simulink model "signal_tranmission"  (R2024b)
settings: Solver=ode45  StartTime=0.0  StopTime=10  FixedStep=0.000125  RelTol=1e-3
libraries: dspfdesign x500, commchan3 x1
(part 3 of 7)

== system signal_tranmission/SSB Demod92 ==
  Input Signal : Inport
  Analog Filter Design1 : dspfdesign/Analog Filter Design  method=Butterworth  filttype=Lowpass  N=4  Wlo=5*2*pi  Whi=102*2*pi  Rp=2  Rs=40
  Balanced Modulator1 : Subsystem
  carrier signal : Sin  Frequency=468*2*pi  SampleTime=0
  Out1 : Outport
  wires:
  Analog Filter Design1/1 -> Out1/1
  Balanced Modulator1/1(DSBSC) -> Analog Filter Design1/1
  carrier signal/1 -> Balanced Modulator1/2(Carrier Signal)
  Input Signal/1 -> Balanced Modulator1/1(Input Signal)

== system signal_tranmission/SSB Demod93 ==
  Input Signal : Inport
  Analog Filter Design1 : dspfdesign/Analog Filter Design  method=Butterworth  filttype=Lowpass  N=4  Wlo=5*2*pi  Whi=102*2*pi  Rp=2  Rs=40
  Balanced Modulator1 : Subsystem
  carrier signal : Sin  Frequency=472*2*pi  SampleTime=0
  Out1 : Outport
  wires:
  Analog Filter Design1/1 -> Out1/1
  Balanced Modulator1/1(DSBSC) -> Analog Filter Design1/1
  carrier signal/1 -> Balanced Modulator1/2(Carrier Signal)
  Input Signal/1 -> Balanced Modulator1/1(Input Signal)

== system signal_tranmission/SSB Demod94 ==
  Input Signal : Inport
  Analog Filter Design1 : dspfdesign/Analog Filter Design  method=Butterworth  filttype=Lowpass  N=4  Wlo=5*2*pi  Whi=102*2*pi  Rp=2  Rs=40
  Balanced Modulator1 : Subsystem
  carrier signal : Sin  Frequency=476*2*pi  SampleTime=0
  Out1 : Outport
  wires:
  Analog Filter Design1/1 -> Out1/1
  Balanced Modulator1/1(DSBSC) -> Analog Filter Design1/1
  carrier signal/1 -> Balanced Modulator1/2(Carrier Signal)
  Input Signal/1 -> Balanced Modulator1/1(Input Signal)

== system signal_tranmission/SSB Demod95 ==
  Input Signal : Inport
  Analog Filter Design1 : dspfdesign/Analog Filter Design  method=Butterworth  filttype=Lowpass  N=4  Wlo=5*2*pi  Whi=102*2*pi  Rp=2  Rs=40
  Balanced Modulator1 : Subsystem
  carrier signal : Sin  Frequency=480*2*pi  SampleTime=0
  Out1 : Outport
  wires:
  Analog Filter Design1/1 -> Out1/1
  Balanced Modulator1/1(DSBSC) -> Analog Filter Design1/1
  carrier signal/1 -> Balanced Modulator1/2(Carrier Signal)
  Input Signal/1 -> Balanced Modulator1/1(Input Signal)

== system signal_tranmission/SSB Demod96 ==
  Input Signal : Inport
  Analog Filter Design1 : dspfdesign/Analog Filter Design  method=Butterworth  filttype=Lowpass  N=4  Wlo=5*2*pi  Whi=102*2*pi  Rp=2  Rs=40
  Balanced Modulator1 : Subsystem
  carrier signal : Sin  Frequency=484*2*pi  SampleTime=0
  Out1 : Outport
  wires:
  Analog Filter Design1/1 -> Out1/1
  Balanced Modulator1/1(DSBSC) -> Analog Filter Design1/1
  carrier signal/1 -> Balanced Modulator1/2(Carrier Signal)
  Input Signal/1 -> Balanced Modulator1/1(Input Signal)

== system signal_tranmission/SSB Demod97 ==
  Input Signal : Inport
  Analog Filter Design1 : dspfdesign/Analog Filter Design  method=Butterworth  filttype=Lowpass  N=4  Wlo=5*2*pi  Whi=102*2*pi  Rp=2  Rs=40
  Balanced Modulator1 : Subsystem
  carrier signal : Sin  Frequency=488*2*pi  SampleTime=0
  Out1 : Outport
  wires:
  Analog Filter Design1/1 -> Out1/1
  Balanced Modulator1/1(DSBSC) -> Analog Filter Design1/1
  carrier signal/1 -> Balanced Modulator1/2(Carrier Signal)
  Input Signal/1 -> Balanced Modulator1/1(Input Signal)

== system signal_tranmission/SSB Demod98 ==
  Input Signal : Inport
  Analog Filter Design1 : dspfdesign/Analog Filter Design  method=Butterworth  filttype=Lowpass  N=4  Wlo=5*2*pi  Whi=102*2*pi  Rp=2  Rs=40
  Balanced Modulator1 : Subsystem
  carrier signal : Sin  Frequency=492*2*pi  SampleTime=0
  Out1 : Outport
  wires:
  Analog Filter Design1/1 -> Out1/1
  Balanced Modulator1/1(DSBSC) -> Analog Filter Design1/1
  carrier signal/1 -> Balanced Modulator1/2(Carrier Signal)
  Input Signal/1 -> Balanced Modulator1/1(Input Signal)

== system signal_tranmission/SSB Demod99 ==
  Input Signal : Inport
  Analog Filter Design1 : dspfdesign/Analog Filter Design  method=Butterworth  filttype=Lowpass  N=4  Wlo=5*2*pi  Whi=102*2*pi  Rp=2  Rs=40
  Balanced Modulator1 : Subsystem
  carrier signal : Sin  Frequency=496*2*pi  SampleTime=0
  Out1 : Outport
  wires:
  Analog Filter Design1/1 -> Out1/1
  Balanced Modulator1/1(DSBSC) -> Analog Filter Design1/1
  carrier signal/1 -> Balanced Modulator1/2(Carrier Signal)
  Input Signal/1 -> Balanced Modulator1/1(Input Signal)

== system signal_tranmission/SSB Modulator ==
  Input Signal : Inport
  Analog Filter Design : dspfdesign/Analog Filter Design  method=Butterworth  filttype=Bandpass  N=4  Wlo=98*2*pi  Whi=102*2*pi  Rp=2  Rs=40
  Balanced Modulator : Subsystem
  carrier signal : Sin  Frequency=100*2*pi  SampleTime=0
  Out1 : Outport
  wires:
  carrier signal/1 -> Balanced Modulator/2(Carrier Signal)
  Balanced Modulator/1(DSBSC) -> Analog Filter Design/1
  Analog Filter Design/1 -> Out1/1
  Input Signal/1 -> Balanced Modulator/1(Input Signal)

== system signal_tranmission/SSB Modulator1 ==
  Input Signal : Inport
  Analog Filter Design : dspfdesign/Analog Filter Design  method=Butterworth  filttype=Bandpass  N=4  Wlo=102*2*pi  Whi=106*2*pi  Rp=2  Rs=40
  Balanced Modulator : Subsystem
  carrier signal : Sin  Frequency=104*2*pi  SampleTime=0
  Out1 : Outport
  wires:
  carrier signal/1 -> Balanced Modulator/2(Carrier Signal)
  Balanced Modulator/1(DSBSC) -> Analog Filter Design/1
  Analog Filter Design/1 -> Out1/1
  Input Signal/1 -> Balanced Modulator/1(Input Signal)

== system signal_tranmission/SSB Modulator10 ==
  Input Signal : Inport
  Analog Filter Design : dspfdesign/Analog Filter Design  method=Butterworth  filttype=Bandpass  N=4  Wlo=138*2*pi  Whi=142*2*pi  Rp=2  Rs=40
  Balanced Modulator : Subsystem
  carrier signal : Sin  Frequency=140*2*pi  SampleTime=0
  Out1 : Outport
  wires:
  carrier signal/1 -> Balanced Modulator/2(Carrier Signal)
  Balanced Modulator/1(DSBSC) -> Analog Filter Design/1
  Analog Filter Design/1 -> Out1/1
  Input Signal/1 -> Balanced Modulator/1(Input Signal)

== system signal_tranmission/SSB Modulator11 ==
  Input Signal : Inport
  Analog Filter Design : dspfdesign/Analog Filter Design  method=Butterworth  filttype=Bandpass  N=4  Wlo=142*2*pi  Whi=146*2*pi  Rp=2  Rs=40
  Balanced Modulator : Subsystem
  carrier signal : Sin  Frequency=144*2*pi  SampleTime=0
  Out1 : Outport
  wires:
  carrier signal/1 -> Balanced Modulator/2(Carrier Signal)
  Balanced Modulator/1(DSBSC) -> Analog Filter Design/1
  Analog Filter Design/1 -> Out1/1
  Input Signal/1 -> Balanced Modulator/1(Input Signal)

== system signal_tranmission/SSB Modulator12 ==
  Input Signal : Inport
  Analog Filter Design : dspfdesign/Analog Filter Design  method=Butterworth  filttype=Bandpass  N=4  Wlo=146*2*pi  Whi=150*2*pi  Rp=2  Rs=40
  Balanced Modulator : Subsystem
  carrier signal : Sin  Frequency=148*2*pi  SampleTime=0
  Out1 : Outport
  wires:
  carrier signal/1 -> Balanced Modulator/2(Carrier Signal)
  Balanced Modulator/1(DSBSC) -> Analog Filter Design/1
  Analog Filter Design/1 -> Out1/1
  Input Signal/1 -> Balanced Modulator/1(Input Signal)

== system signal_tranmission/SSB Modulator13 ==
  Input Signal : Inport
  Analog Filter Design : dspfdesign/Analog Filter Design  method=Butterworth  filttype=Bandpass  N=4  Wlo=150*2*pi  Whi=154*2*pi  Rp=2  Rs=40
  Balanced Modulator : Subsystem
  carrier signal : Sin  Frequency=152*2*pi  SampleTime=0
  Out1 : Outport
  wires:
  carrier signal/1 -> Balanced Modulator/2(Carrier Signal)
  Balanced Modulator/1(DSBSC) -> Analog Filter Design/1
  Analog Filter Design/1 -> Out1/1
  Input Signal/1 -> Balanced Modulator/1(Input Signal)

== system signal_tranmission/SSB Modulator14 ==
  Input Signal : Inport
  Analog Filter Design : dspfdesign/Analog Filter Design  method=Butterworth  filttype=Bandpass  N=4  Wlo=154*2*pi  Whi=158*2*pi  Rp=2  Rs=40
  Balanced Modulator : Subsystem
  carrier signal : Sin  Frequency=156*2*pi  SampleTime=0
  Out1 : Outport
  wires:
  carrier signal/1 -> Balanced Modulator/2(Carrier Signal)
  Balanced Modulator/1(DSBSC) -> Analog Filter Design/1
  Analog Filter Design/1 -> Out1/1
  Input Signal/1 -> Balanced Modulator/1(Input Signal)

== system signal_tranmission/SSB Modulator15 ==
  Input Signal : Inport
  Analog Filter Design : dspfdesign/Analog Filter Design  method=Butterworth  filttype=Bandpass  N=4  Wlo=158*2*pi  Whi=162*2*pi  Rp=2  Rs=40
  Balanced Modulator : Subsystem
  carrier signal : Sin  Frequency=160*2*pi  SampleTime=0
  Out1 : Outport
  wires:
  carrier signal/1 -> Balanced Modulator/2(Carrier Signal)
  Balanced Modulator/1(DSBSC) -> Analog Filter Design/1
  Analog Filter Design/1 -> Out1/1
  Input Signal/1 -> Balanced Modulator/1(Input Signal)

== system signal_tranmission/SSB Modulator16 ==
  Input Signal : Inport
  Analog Filter Design : dspfdesign/Analog Filter Design  method=Butterworth  filttype=Bandpass  N=4  Wlo=162*2*pi  Whi=166*2*pi  Rp=2  Rs=40
  Balanced Modulator : Subsystem
  carrier signal : Sin  Frequency=164*2*pi  SampleTime=0
  Out1 : Outport
  wires:
  carrier signal/1 -> Balanced Modulator/2(Carrier Signal)
  Balanced Modulator/1(DSBSC) -> Analog Filter Design/1
  Analog Filter Design/1 -> Out1/1
  Input Signal/1 -> Balanced Modulator/1(Input Signal)

== system signal_tranmission/SSB Modulator17 ==
  Input Signal : Inport
  Analog Filter Design : dspfdesign/Analog Filter Design  method=Butterworth  filttype=Bandpass  N=4  Wlo=166*2*pi  Whi=170*2*pi  Rp=2  Rs=40
  Balanced Modulator : Subsystem
  carrier signal : Sin  Frequency=168*2*pi  SampleTime=0
  Out1 : Outport
  wires:
  carrier signal/1 -> Balanced Modulator/2(Carrier Signal)
  Balanced Modulator/1(DSBSC) -> Analog Filter Design/1
  Analog Filter Design/1 -> Out1/1
  Input Signal/1 -> Balanced Modulator/1(Input Signal)

== system signal_tranmission/SSB Modulator18 ==
  Input Signal : Inport
  Analog Filter Design : dspfdesign/Analog Filter Design  method=Butterworth  filttype=Bandpass  N=4  Wlo=170*2*pi  Whi=174*2*pi  Rp=2  Rs=40
  Balanced Modulator : Subsystem
  carrier signal : Sin  Frequency=172*2*pi  SampleTime=0
  Out1 : Outport
  wires:
  carrier signal/1 -> Balanced Modulator/2(Carrier Signal)
  Balanced Modulator/1(DSBSC) -> Analog Filter Design/1
  Analog Filter Design/1 -> Out1/1
  Input Signal/1 -> Balanced Modulator/1(Input Signal)

== system signal_tranmission/SSB Modulator19 ==
  Input Signal : Inport
  Analog Filter Design : dspfdesign/Analog Filter Design  method=Butterworth  filttype=Bandpass  N=4  Wlo=174*2*pi  Whi=178*2*pi  Rp=2  Rs=40
  Balanced Modulator : Subsystem
  carrier signal : Sin  Frequency=176*2*pi  SampleTime=0
  Out1 : Outport
  wires:
  carrier signal/1 -> Balanced Modulator/2(Carrier Signal)
  Balanced Modulator/1(DSBSC) -> Analog Filter Design/1
  Analog Filter Design/1 -> Out1/1
  Input Signal/1 -> Balanced Modulator/1(Input Signal)

== system signal_tranmission/SSB Modulator2 ==
  Input Signal : Inport
  Analog Filter Design : dspfdesign/Analog Filter Design  method=Butterworth  filttype=Bandpass  N=4  Wlo=106*2*pi  Whi=110*2*pi  Rp=2  Rs=40
  Balanced Modulator : Subsystem
  carrier signal : Sin  Frequency=108*2*pi  SampleTime=0
  Out1 : Outport
  wires:
  carrier signal/1 -> Balanced Modulator/2(Carrier Signal)
  Balanced Modulator/1(DSBSC) -> Analog Filter Design/1
  Analog Filter Design/1 -> Out1/1
  Input Signal/1 -> Balanced Modulator/1(Input Signal)

== system signal_tranmission/SSB Modulator20 ==
  Input Signal : Inport
  Analog Filter Design : dspfdesign/Analog Filter Design  method=Butterworth  filttype=Bandpass  N=4  Wlo=178*2*pi  Whi=182*2*pi  Rp=2  Rs=40
  Balanced Modulator : Subsystem
  carrier signal : Sin  Frequency=180*2*pi  SampleTime=0
  Out1 : Outport
  wires:
  carrier signal/1 -> Balanced Modulator/2(Carrier Signal)
  Balanced Modulator/1(DSBSC) -> Analog Filter Design/1
  Analog Filter Design/1 -> Out1/1
  Input Signal/1 -> Balanced Modulator/1(Input Signal)

== system signal_tranmission/SSB Modulator21 ==
  Input Signal : Inport
  Analog Filter Design : dspfdesign/Analog Filter Design  method=Butterworth  filttype=Bandpass  N=4  Wlo=182*2*pi  Whi=186*2*pi  Rp=2  Rs=40
  Balanced Modulator : Subsystem
  carrier signal : Sin  Frequency=184*2*pi  SampleTime=0
  Out1 : Outport
  wires:
  carrier signal/1 -> Balanced Modulator/2(Carrier Signal)
  Balanced Modulator/1(DSBSC) -> Analog Filter Design/1
  Analog Filter Design/1 -> Out1/1
  Input Signal/1 -> Balanced Modulator/1(Input Signal)

== system signal_tranmission/SSB Modulator22 ==
  Input Signal : Inport
  Analog Filter Design : dspfdesign/Analog Filter Design  method=Butterworth  filttype=Bandpass  N=4  Wlo=186*2*pi  Whi=190*2*pi  Rp=2  Rs=40
  Balanced Modulator : Subsystem
  carrier signal : Sin  Frequency=188*2*pi  SampleTime=0
  Out1 : Outport
  wires:
  carrier signal/1 -> Balanced Modulator/2(Carrier Signal)
  Balanced Modulator/1(DSBSC) -> Analog Filter Design/1
  Analog Filter Design/1 -> Out1/1
  Input Signal/1 -> Balanced Modulator/1(Input Signal)

== system signal_tranmission/SSB Modulator23 ==
  Input Signal : Inport
  Analog Filter Design : dspfdesign/Analog Filter Design  method=Butterworth  filttype=Bandpass  N=4  Wlo=190*2*pi  Whi=194*2*pi  Rp=2  Rs=40
  Balanced Modulator : Subsystem
  carrier signal : Sin  Frequency=192*2*pi  SampleTime=0
  Out1 : Outport
  wires:
  carrier signal/1 -> Balanced Modulator/2(Carrier Signal)
  Balanced Modulator/1(DSBSC) -> Analog Filter Design/1
  Analog Filter Design/1 -> Out1/1
  Input Signal/1 -> Balanced Modulator/1(Input Signal)

== system signal_tranmission/SSB Modulator24 ==
  Input Signal : Inport
  Analog Filter Design : dspfdesign/Analog Filter Design  method=Butterworth  filttype=Bandpass  N=4  Wlo=194*2*pi  Whi=198*2*pi  Rp=2  Rs=40
  Balanced Modulator : Subsystem
  carrier signal : Sin  Frequency=196*2*pi  SampleTime=0
  Out1 : Outport
  wires:
  carrier signal/1 -> Balanced Modulator/2(Carrier Signal)
  Balanced Modulator/1(DSBSC) -> Analog Filter Design/1
  Analog Filter Design/1 -> Out1/1
  Input Signal/1 -> Balanced Modulator/1(Input Signal)

== system signal_tranmission/SSB Modulator25 ==
  Input Signal : Inport
  Analog Filter Design : dspfdesign/Analog Filter Design  method=Butterworth  filttype=Bandpass  N=4  Wlo=198*2*pi  Whi=202*2*pi  Rp=2  Rs=40
  Balanced Modulator : Subsystem
  carrier signal : Sin  Frequency=200*2*pi  SampleTime=0
  Out1 : Outport
  wires:
  carrier signal/1 -> Balanced Modulator/2(Carrier Signal)
  Balanced Modulator/1(DSBSC) -> Analog Filter Design/1
  Analog Filter Design/1 -> Out1/1
  Input Signal/1 -> Balanced Modulator/1(Input Signal)

== system signal_tranmission/SSB Modulator26 ==
  Input Signal : Inport
  Analog Filter Design : dspfdesign/Analog Filter Design  method=Butterworth  filttype=Bandpass  N=4  Wlo=202*2*pi  Whi=206*2*pi  Rp=2  Rs=40
  Balanced Modulator : Subsystem
  carrier signal : Sin  Frequency=204*2*pi  SampleTime=0
  Out1 : Outport
  wires:
  carrier signal/1 -> Balanced Modulator/2(Carrier Signal)
  Balanced Modulator/1(DSBSC) -> Analog Filter Design/1
  Analog Filter Design/1 -> Out1/1
  Input Signal/1 -> Balanced Modulator/1(Input Signal)

== system signal_tranmission/SSB Modulator27 ==
  Input Signal : Inport
  Analog Filter Design : dspfdesign/Analog Filter Design  method=Butterworth  filttype=Bandpass  N=4  Wlo=206*2*pi  Whi=210*2*pi  Rp=2  Rs=40
  Balanced Modulator : Subsystem
  carrier signal : Sin  Frequency=208*2*pi  SampleTime=0
  Out1 : Outport
  wires:
  carrier signal/1 -> Balanced Modulator/2(Carrier Signal)
  Balanced Modulator/1(DSBSC) -> Analog Filter Design/1
  Analog Filter Design/1 -> Out1/1
  Input Signal/1 -> Balanced Modulator/1(Input Signal)

== system signal_tranmission/SSB Modulator28 ==
  Input Signal : Inport
  Analog Filter Design : dspfdesign/Analog Filter Design  method=Butterworth  filttype=Bandpass  N=4  Wlo=210*2*pi  Whi=214*2*pi  Rp=2  Rs=40
  Balanced Modulator : Subsystem
  carrier signal : Sin  Frequency=212*2*pi  SampleTime=0
  Out1 : Outport
  wires:
  carrier signal/1 -> Balanced Modulator/2(Carrier Signal)
  Balanced Modulator/1(DSBSC) -> Analog Filter Design/1
  Analog Filter Design/1 -> Out1/1
  Input Signal/1 -> Balanced Modulator/1(Input Signal)

== system signal_tranmission/SSB Modulator29 ==
  Input Signal : Inport
  Analog Filter Design : dspfdesign/Analog Filter Design  method=Butterworth  filttype=Bandpass  N=4  Wlo=214*2*pi  Whi=218*2*pi  Rp=2  Rs=40
  Balanced Modulator : Subsystem
  carrier signal : Sin  Frequency=216*2*pi  SampleTime=0
  Out1 : Outport
  wires:
  carrier signal/1 -> Balanced Modulator/2(Carrier Signal)
  Balanced Modulator/1(DSBSC) -> Analog Filter Design/1
  Analog Filter Design/1 -> Out1/1
  Input Signal/1 -> Balanced Modulator/1(Input Signal)

== system signal_tranmission/SSB Modulator3 ==
  Input Signal : Inport
  Analog Filter Design : dspfdesign/Analog Filter Design  method=Butterworth  filttype=Bandpass  N=4  Wlo=110*2*pi  Whi=114*2*pi  Rp=2  Rs=40
  Balanced Modulator : Subsystem
  carrier signal : Sin  Frequency=112*2*pi  SampleTime=0
  Out1 : Outport
  wires:
  carrier signal/1 -> Balanced Modulator/2(Carrier Signal)
  Balanced Modulator/1(DSBSC) -> Analog Filter Design/1
  Analog Filter Design/1 -> Out1/1
  Input Signal/1 -> Balanced Modulator/1(Input Signal)

== system signal_tranmission/SSB Modulator30 ==
  Input Signal : Inport
  Analog Filter Design : dspfdesign/Analog Filter Design  method=Butterworth  filttype=Bandpass  N=4  Wlo=218*2*pi  Whi=222*2*pi  Rp=2  Rs=40
  Balanced Modulator : Subsystem
  carrier signal : Sin  Frequency=220*2*pi  SampleTime=0
  Out1 : Outport
  wires:
  carrier signal/1 -> Balanced Modulator/2(Carrier Signal)
  Balanced Modulator/1(DSBSC) -> Analog Filter Design/1
  Analog Filter Design/1 -> Out1/1
  Input Signal/1 -> Balanced Modulator/1(Input Signal)

== system signal_tranmission/SSB Modulator31 ==
  Input Signal : Inport
  Analog Filter Design : dspfdesign/Analog Filter Design  method=Butterworth  filttype=Bandpass  N=4  Wlo=222*2*pi  Whi=226*2*pi  Rp=2  Rs=40
  Balanced Modulator : Subsystem
  carrier signal : Sin  Frequency=224*2*pi  SampleTime=0
  Out1 : Outport
  wires:
  carrier signal/1 -> Balanced Modulator/2(Carrier Signal)
  Balanced Modulator/1(DSBSC) -> Analog Filter Design/1
  Analog Filter Design/1 -> Out1/1
  Input Signal/1 -> Balanced Modulator/1(Input Signal)

== system signal_tranmission/SSB Modulator32 ==
  Input Signal : Inport
  Analog Filter Design : dspfdesign/Analog Filter Design  method=Butterworth  filttype=Bandpass  N=4  Wlo=226*2*pi  Whi=230*2*pi  Rp=2  Rs=40
  Balanced Modulator : Subsystem
  carrier signal : Sin  Frequency=228*2*pi  SampleTime=0
  Out1 : Outport
  wires:
  carrier signal/1 -> Balanced Modulator/2(Carrier Signal)
  Balanced Modulator/1(DSBSC) -> Analog Filter Design/1
  Analog Filter Design/1 -> Out1/1
  Input Signal/1 -> Balanced Modulator/1(Input Signal)

== system signal_tranmission/SSB Modulator33 ==
  Input Signal : Inport
  Analog Filter Design : dspfdesign/Analog Filter Design  method=Butterworth  filttype=Bandpass  N=4  Wlo=230*2*pi  Whi=234*2*pi  Rp=2  Rs=40
  Balanced Modulator : Subsystem
  carrier signal : Sin  Frequency=232*2*pi  SampleTime=0
  Out1 : Outport
  wires:
  carrier signal/1 -> Balanced Modulator/2(Carrier Signal)
  Balanced Modulator/1(DSBSC) -> Analog Filter Design/1
  Analog Filter Design/1 -> Out1/1
  Input Signal/1 -> Balanced Modulator/1(Input Signal)

== system signal_tranmission/SSB Modulator34 ==
  Input Signal : Inport
  Analog Filter Design : dspfdesign/Analog Filter Design  method=Butterworth  filttype=Bandpass  N=4  Wlo=234*2*pi  Whi=238*2*pi  Rp=2  Rs=40
  Balanced Modulator : Subsystem
  carrier signal : Sin  Frequency=236*2*pi  SampleTime=0
  Out1 : Outport
  wires:
  carrier signal/1 -> Balanced Modulator/2(Carrier Signal)
  Balanced Modulator/1(DSBSC) -> Analog Filter Design/1
  Analog Filter Design/1 -> Out1/1
  Input Signal/1 -> Balanced Modulator/1(Input Signal)

== system signal_tranmission/SSB Modulator35 ==
  Input Signal : Inport
  Analog Filter Design : dspfdesign/Analog Filter Design  method=Butterworth  filttype=Bandpass  N=4  Wlo=238*2*pi  Whi=242*2*pi  Rp=2  Rs=40
  Balanced Modulator : Subsystem
  carrier signal : Sin  Frequency=240*2*pi  SampleTime=0
  Out1 : Outport
  wires:
  carrier signal/1 -> Balanced Modulator/2(Carrier Signal)
  Balanced Modulator/1(DSBSC) -> Analog Filter Design/1
  Analog Filter Design/1 -> Out1/1
  Input Signal/1 -> Balanced Modulator/1(Input Signal)

== system signal_tranmission/SSB Modulator36 ==
  Input Signal : Inport
  Analog Filter Design : dspfdesign/Analog Filter Design  method=Butterworth  filttype=Bandpass  N=4  Wlo=242*2*pi  Whi=246*2*pi  Rp=2  Rs=40
  Balanced Modulator : Subsystem
  carrier signal : Sin  Frequency=244*2*pi  SampleTime=0
  Out1 : Outport
  wires:
  carrier signal/1 -> Balanced Modulator/2(Carrier Signal)
  Balanced Modulator/1(DSBSC) -> Analog Filter Design/1
  Analog Filter Design/1 -> Out1/1
  Input Signal/1 -> Balanced Modulator/1(Input Signal)

== system signal_tranmission/SSB Modulator37 ==
  Input Signal : Inport
  Analog Filter Design : dspfdesign/Analog Filter Design  method=Butterworth  filttype=Bandpass  N=4  Wlo=246*2*pi  Whi=250*2*pi  Rp=2  Rs=40
  Balanced Modulator : Subsystem
  carrier signal : Sin  Frequency=248*2*pi  SampleTime=0
  Out1 : Outport
  wires:
  carrier signal/1 -> Balanced Modulator/2(Carrier Signal)
  Balanced Modulator/1(DSBSC) -> Analog Filter Design/1
  Analog Filter Design/1 -> Out1/1
  Input Signal/1 -> Balanced Modulator/1(Input Signal)

== system signal_tranmission/SSB Modulator38 ==
  Input Signal : Inport
  Analog Filter Design : dspfdesign/Analog Filter Design  method=Butterworth  filttype=Bandpass  N=4  Wlo=250*2*pi  Whi=254*2*pi  Rp=2  Rs=40
  Balanced Modulator : Subsystem
  carrier signal : Sin  Frequency=252*2*pi  SampleTime=0
  Out1 : Outport
  wires:
  carrier signal/1 -> Balanced Modulator/2(Carrier Signal)
  Balanced Modulator/1(DSBSC) -> Analog Filter Design/1
  Analog Filter Design/1 -> Out1/1
  Input Signal/1 -> Balanced Modulator/1(Input Signal)

== system signal_tranmission/SSB Modulator39 ==
  Input Signal : Inport
  Analog Filter Design : dspfdesign/Analog Filter Design  method=Butterworth  filttype=Bandpass  N=4  Wlo=254*2*pi  Whi=258*2*pi  Rp=2  Rs=40
  Balanced Modulator : Subsystem
  carrier signal : Sin  Frequency=256*2*pi  SampleTime=0
  Out1 : Outport
  wires:
  carrier signal/1 -> Balanced Modulator/2(Carrier Signal)
  Balanced Modulator/1(DSBSC) -> Analog Filter Design/1
  Analog Filter Design/1 -> Out1/1
  Input Signal/1 -> Balanced Modulator/1(Input Signal)

== system signal_tranmission/SSB Modulator4 ==
  Input Signal : Inport
  Analog Filter Design : dspfdesign/Analog Filter Design  method=Butterworth  filttype=Bandpass  N=4  Wlo=114*2*pi  Whi=118*2*pi  Rp=2  Rs=40
  Balanced Modulator : Subsystem
  carrier signal : Sin  Frequency=116*2*pi  SampleTime=0
  Out1 : Outport
  wires:
  carrier signal/1 -> Balanced Modulator/2(Carrier Signal)
  Balanced Modulator/1(DSBSC) -> Analog Filter Design/1
  Analog Filter Design/1 -> Out1/1
  Input Signal/1 -> Balanced Modulator/1(Input Signal)

== system signal_tranmission/SSB Modulator40 ==
  Input Signal : Inport
  Analog Filter Design : dspfdesign/Analog Filter Design  method=Butterworth  filttype=Bandpass  N=4  Wlo=258*2*pi  Whi=262*2*pi  Rp=2  Rs=40
  Balanced Modulator : Subsystem
  carrier signal : Sin  Frequency=260*2*pi  SampleTime=0
  Out1 : Outport
  wires:
  carrier signal/1 -> Balanced Modulator/2(Carrier Signal)
  Balanced Modulator/1(DSBSC) -> Analog Filter Design/1
  Analog Filter Design/1 -> Out1/1
  Input Signal/1 -> Balanced Modulator/1(Input Signal)

== system signal_tranmission/SSB Modulator41 ==
  Input Signal : Inport
  Analog Filter Design : dspfdesign/Analog Filter Design  method=Butterworth  filttype=Bandpass  N=4  Wlo=262*2*pi  Whi=266*2*pi  Rp=2  Rs=40
  Balanced Modulator : Subsystem
  carrier signal : Sin  Frequency=264*2*pi  SampleTime=0
  Out1 : Outport
  wires:
  carrier signal/1 -> Balanced Modulator/2(Carrier Signal)
  Balanced Modulator/1(DSBSC) -> Analog Filter Design/1
  Analog Filter Design/1 -> Out1/1
  Input Signal/1 -> Balanced Modulator/1(Input Signal)

== system signal_tranmission/SSB Modulator42 ==
  Input Signal : Inport
  Analog Filter Design : dspfdesign/Analog Filter Design  method=Butterworth  filttype=Bandpass  N=4  Wlo=266*2*pi  Whi=270*2*pi  Rp=2  Rs=40
  Balanced Modulator : Subsystem
  carrier signal : Sin  Frequency=268*2*pi  SampleTime=0
  Out1 : Outport
  wires:
  carrier signal/1 -> Balanced Modulator/2(Carrier Signal)
  Balanced Modulator/1(DSBSC) -> Analog Filter Design/1
  Analog Filter Design/1 -> Out1/1
  Input Signal/1 -> Balanced Modulator/1(Input Signal)

== system signal_tranmission/SSB Modulator43 ==
  Input Signal : Inport
  Analog Filter Design : dspfdesign/Analog Filter Design  method=Butterworth  filttype=Bandpass  N=4  Wlo=270*2*pi  Whi=274*2*pi  Rp=2  Rs=40
  Balanced Modulator : Subsystem
  carrier signal : Sin  Frequency=272*2*pi  SampleTime=0
  Out1 : Outport
  wires:
  carrier signal/1 -> Balanced Modulator/2(Carrier Signal)
  Balanced Modulator/1(DSBSC) -> Analog Filter Design/1
  Analog Filter Design/1 -> Out1/1
  Input Signal/1 -> Balanced Modulator/1(Input Signal)

== system signal_tranmission/SSB Modulator44 ==
  Input Signal : Inport
  Analog Filter Design : dspfdesign/Analog Filter Design  method=Butterworth  filttype=Bandpass  N=4  Wlo=274*2*pi  Whi=278*2*pi  Rp=2  Rs=40
  Balanced Modulator : Subsystem
  carrier signal : Sin  Frequency=276*2*pi  SampleTime=0
  Out1 : Outport
  wires:
  carrier signal/1 -> Balanced Modulator/2(Carrier Signal)
  Balanced Modulator/1(DSBSC) -> Analog Filter Design/1
  Analog Filter Design/1 -> Out1/1
  Input Signal/1 -> Balanced Modulator/1(Input Signal)

== system signal_tranmission/SSB Modulator45 ==
  Input Signal : Inport
  Analog Filter Design : dspfdesign/Analog Filter Design  method=Butterworth  filttype=Bandpass  N=4  Wlo=278*2*pi  Whi=282*2*pi  Rp=2  Rs=40
  Balanced Modulator : Subsystem
  carrier signal : Sin  Frequency=280*2*pi  SampleTime=0
  Out1 : Outport
  wires:
  carrier signal/1 -> Balanced Modulator/2(Carrier Signal)
  Balanced Modulator/1(DSBSC) -> Analog Filter Design/1
  Analog Filter Design/1 -> Out1/1
  Input Signal/1 -> Balanced Modulator/1(Input Signal)

== system signal_tranmission/SSB Modulator46 ==
  Input Signal : Inport
  Analog Filter Design : dspfdesign/Analog Filter Design  method=Butterworth  filttype=Bandpass  N=4  Wlo=282*2*pi  Whi=286*2*pi  Rp=2  Rs=40
  Balanced Modulator : Subsystem
  carrier signal : Sin  Frequency=284*2*pi  SampleTime=0
  Out1 : Outport
  wires:
  carrier signal/1 -> Balanced Modulator/2(Carrier Signal)
  Balanced Modulator/1(DSBSC) -> Analog Filter Design/1
  Analog Filter Design/1 -> Out1/1
  Input Signal/1 -> Balanced Modulator/1(Input Signal)

== system signal_tranmission/SSB Modulator47 ==
  Input Signal : Inport
  Analog Filter Design : dspfdesign/Analog Filter Design  method=Butterworth  filttype=Bandpass  N=4  Wlo=286*2*pi  Whi=290*2*pi  Rp=2  Rs=40
  Balanced Modulator : Subsystem
  carrier signal : Sin  Frequency=288*2*pi  SampleTime=0
  Out1 : Outport
  wires:
  carrier signal/1 -> Balanced Modulator/2(Carrier Signal)
  Balanced Modulator/1(DSBSC) -> Analog Filter Design/1
  Analog Filter Design/1 -> Out1/1
  Input Signal/1 -> Balanced Modulator/1(Input Signal)

== system signal_tranmission/SSB Modulator48 ==
  Input Signal : Inport
  Analog Filter Design : dspfdesign/Analog Filter Design  method=Butterworth  filttype=Bandpass  N=4  Wlo=290*2*pi  Whi=294*2*pi  Rp=2  Rs=40
  Balanced Modulator : Subsystem
  carrier signal : Sin  Frequency=292*2*pi  SampleTime=0
  Out1 : Outport
  wires:
  carrier signal/1 -> Balanced Modulator/2(Carrier Signal)
  Balanced Modulator/1(DSBSC) -> Analog Filter Design/1
  Analog Filter Design/1 -> Out1/1
  Input Signal/1 -> Balanced Modulator/1(Input Signal)

== system signal_tranmission/SSB Modulator49 ==
  Input Signal : Inport
  Analog Filter Design : dspfdesign/Analog Filter Design  method=Butterworth  filttype=Bandpass  N=4  Wlo=294*2*pi  Whi=298*2*pi  Rp=2  Rs=40
  Balanced Modulator : Subsystem
  carrier signal : Sin  Frequency=296*2*pi  SampleTime=0
  Out1 : Outport
  wires:
  carrier signal/1 -> Balanced Modulator/2(Carrier Signal)
  Balanced Modulator/1(DSBSC) -> Analog Filter Design/1
  Analog Filter Design/1 -> Out1/1
  Input Signal/1 -> Balanced Modulator/1(Input Signal)

== system signal_tranmission/SSB Modulator5 ==
  Input Signal : Inport
  Analog Filter Design : dspfdesign/Analog Filter Design  method=Butterworth  filttype=Bandpass  N=4  Wlo=118*2*pi  Whi=122*2*pi  Rp=2  Rs=40
  Balanced Modulator : Subsystem
  carrier signal : Sin  Frequency=120*2*pi  SampleTime=0
  Out1 : Outport
  wires:
  carrier signal/1 -> Balanced Modulator/2(Carrier Signal)
  Balanced Modulator/1(DSBSC) -> Analog Filter Design/1
  Analog Filter Design/1 -> Out1/1
  Input Signal/1 -> Balanced Modulator/1(Input Signal)

== system signal_tranmission/SSB Modulator50 ==
  Input Signal : Inport
  Analog Filter Design : dspfdesign/Analog Filter Design  method=Butterworth  filttype=Bandpass  N=4  Wlo=298*2*pi  Whi=302*2*pi  Rp=2  Rs=40
  Balanced Modulator : Subsystem
  carrier signal : Sin  Frequency=300*2*pi  SampleTime=0
  Out1 : Outport
  wires:
  carrier signal/1 -> Balanced Modulator/2(Carrier Signal)
  Balanced Modulator/1(DSBSC) -> Analog Filter Design/1
  Analog Filter Design/1 -> Out1/1
  Input Signal/1 -> Balanced Modulator/1(Input Signal)

== system signal_tranmission/SSB Modulator51 ==
  Input Signal : Inport
  Analog Filter Design : dspfdesign/Analog Filter Design  method=Butterworth  filttype=Bandpass  N=4  Wlo=302*2*pi  Whi=306*2*pi  Rp=2  Rs=40
  Balanced Modulator : Subsystem
  carrier signal : Sin  Frequency=304*2*pi  SampleTime=0
  Out1 : Outport
  wires:
  carrier signal/1 -> Balanced Modulator/2(Carrier Signal)
  Balanced Modulator/1(DSBSC) -> Analog Filter Design/1
  Analog Filter Design/1 -> Out1/1
  Input Signal/1 -> Balanced Modulator/1(Input Signal)

== system signal_tranmission/SSB Modulator52 ==
  Input Signal : Inport
  Analog Filter Design : dspfdesign/Analog Filter Design  method=Butterworth  filttype=Bandpass  N=4  Wlo=306*2*pi  Whi=310*2*pi  Rp=2  Rs=40
  Balanced Modulator : Subsystem
  carrier signal : Sin  Frequency=308*2*pi  SampleTime=0
  Out1 : Outport
  wires:
  carrier signal/1 -> Balanced Modulator/2(Carrier Signal)
  Balanced Modulator/1(DSBSC) -> Analog Filter Design/1
  Analog Filter Design/1 -> Out1/1
  Input Signal/1 -> Balanced Modulator/1(Input Signal)

== system signal_tranmission/SSB Modulator53 ==
  Input Signal : Inport
  Analog Filter Design : dspfdesign/Analog Filter Design  method=Butterworth  filttype=Bandpass  N=4  Wlo=310*2*pi  Whi=314*2*pi  Rp=2  Rs=40
  Balanced Modulator : Subsystem
  carrier signal : Sin  Frequency=312*2*pi  SampleTime=0
  Out1 : Outport
  wires:
  carrier signal/1 -> Balanced Modulator/2(Carrier Signal)
  Balanced Modulator/1(DSBSC) -> Analog Filter Design/1
  Analog Filter Design/1 -> Out1/1
  Input Signal/1 -> Balanced Modulator/1(Input Signal)

== system signal_tranmission/SSB Modulator54 ==
  Input Signal : Inport
  Analog Filter Design : dspfdesign/Analog Filter Design  method=Butterworth  filttype=Bandpass  N=4  Wlo=314*2*pi  Whi=318*2*pi  Rp=2  Rs=40
  Balanced Modulator : Subsystem
  carrier signal : Sin  Frequency=316*2*pi  SampleTime=0
  Out1 : Outport
  wires:
  carrier signal/1 -> Balanced Modulator/2(Carrier Signal)
  Balanced Modulator/1(DSBSC) -> Analog Filter Design/1
  Analog Filter Design/1 -> Out1/1
  Input Signal/1 -> Balanced Modulator/1(Input Signal)

== system signal_tranmission/SSB Modulator55 ==
  Input Signal : Inport
  Analog Filter Design : dspfdesign/Analog Filter Design  method=Butterworth  filttype=Bandpass  N=4  Wlo=318*2*pi  Whi=322*2*pi  Rp=2  Rs=40
  Balanced Modulator : Subsystem
  carrier signal : Sin  Frequency=320*2*pi  SampleTime=0
  Out1 : Outport
  wires:
  carrier signal/1 -> Balanced Modulator/2(Carrier Signal)
  Balanced Modulator/1(DSBSC) -> Analog Filter Design/1
  Analog Filter Design/1 -> Out1/1
  Input Signal/1 -> Balanced Modulator/1(Input Signal)

== system signal_tranmission/SSB Modulator56 ==
  Input Signal : Inport
  Analog Filter Design : dspfdesign/Analog Filter Design  method=Butterworth  filttype=Bandpass  N=4  Wlo=322*2*pi  Whi=326*2*pi  Rp=2  Rs=40
  Balanced Modulator : Subsystem
  carrier signal : Sin  Frequency=324*2*pi  SampleTime=0
  Out1 : Outport
  wires:
  carrier signal/1 -> Balanced Modulator/2(Carrier Signal)
  Balanced Modulator/1(DSBSC) -> Analog Filter Design/1
  Analog Filter Design/1 -> Out1/1
  Input Signal/1 -> Balanced Modulator/1(Input Signal)

== system signal_tranmission/SSB Modulator57 ==
  Input Signal : Inport
  Analog Filter Design : dspfdesign/Analog Filter Design  method=Butterworth  filttype=Bandpass  N=4  Wlo=326*2*pi  Whi=330*2*pi  Rp=2  Rs=40
  Balanced Modulator : Subsystem
  carrier signal : Sin  Frequency=328*2*pi  SampleTime=0
  Out1 : Outport
  wires:
  carrier signal/1 -> Balanced Modulator/2(Carrier Signal)
  Balanced Modulator/1(DSBSC) -> Analog Filter Design/1
  Analog Filter Design/1 -> Out1/1
  Input Signal/1 -> Balanced Modulator/1(Input Signal)

== system signal_tranmission/SSB Modulator58 ==
  Input Signal : Inport
  Analog Filter Design : dspfdesign/Analog Filter Design  method=Butterworth  filttype=Bandpass  N=4  Wlo=330*2*pi  Whi=334*2*pi  Rp=2  Rs=40
  Balanced Modulator : Subsystem
  carrier signal : Sin  Frequency=332*2*pi  SampleTime=0
  Out1 : Outport
  wires:
  carrier signal/1 -> Balanced Modulator/2(Carrier Signal)
  Balanced Modulator/1(DSBSC) -> Analog Filter Design/1
  Analog Filter Design/1 -> Out1/1
  Input Signal/1 -> Balanced Modulator/1(Input Signal)

== system signal_tranmission/SSB Modulator59 ==
  Input Signal : Inport
  Analog Filter Design : dspfdesign/Analog Filter Design  method=Butterworth  filttype=Bandpass  N=4  Wlo=334*2*pi  Whi=338*2*pi  Rp=2  Rs=40
  Balanced Modulator : Subsystem
  carrier signal : Sin  Frequency=336*2*pi  SampleTime=0
  Out1 : Outport
  wires:
  carrier signal/1 -> Balanced Modulator/2(Carrier Signal)
  Balanced Modulator/1(DSBSC) -> Analog Filter Design/1
  Analog Filter Design/1 -> Out1/1
  Input Signal/1 -> Balanced Modulator/1(Input Signal)

== system signal_tranmission/SSB Modulator6 ==
  Input Signal : Inport
  Analog Filter Design : dspfdesign/Analog Filter Design  method=Butterworth  filttype=Bandpass  N=4  Wlo=122*2*pi  Whi=126*2*pi  Rp=2  Rs=40
  Balanced Modulator : Subsystem
  carrier signal : Sin  Frequency=124*2*pi  SampleTime=0
  Out1 : Outport
  wires:
  carrier signal/1 -> Balanced Modulator/2(Carrier Signal)
  Balanced Modulator/1(DSBSC) -> Analog Filter Design/1
  Analog Filter Design/1 -> Out1/1
  Input Signal/1 -> Balanced Modulator/1(Input Signal)

== system signal_tranmission/SSB Modulator60 ==
  Input Signal : Inport
  Analog Filter Design : dspfdesign/Analog Filter Design  method=Butterworth  filttype=Bandpass  N=4  Wlo=338*2*pi  Whi=342*2*pi  Rp=2  Rs=40
  Balanced Modulator : Subsystem
  carrier signal : Sin  Frequency=340*2*pi  SampleTime=0
  Out1 : Outport
  wires:
  carrier signal/1 -> Balanced Modulator/2(Carrier Signal)
  Balanced Modulator/1(DSBSC) -> Analog Filter Design/1
  Analog Filter Design/1 -> Out1/1
  Input Signal/1 -> Balanced Modulator/1(Input Signal)

== system signal_tranmission/SSB Modulator61 ==
  Input Signal : Inport
  Analog Filter Design : dspfdesign/Analog Filter Design  method=Butterworth  filttype=Bandpass  N=4  Wlo=342*2*pi  Whi=346*2*pi  Rp=2  Rs=40
  Balanced Modulator : Subsystem
  carrier signal : Sin  Frequency=344*2*pi  SampleTime=0
  Out1 : Outport
  wires:
  carrier signal/1 -> Balanced Modulator/2(Carrier Signal)
  Balanced Modulator/1(DSBSC) -> Analog Filter Design/1
  Analog Filter Design/1 -> Out1/1
  Input Signal/1 -> Balanced Modulator/1(Input Signal)

== system signal_tranmission/SSB Modulator62 ==
  Input Signal : Inport
  Analog Filter Design : dspfdesign/Analog Filter Design  method=Butterworth  filttype=Bandpass  N=4  Wlo=346*2*pi  Whi=350*2*pi  Rp=2  Rs=40
  Balanced Modulator : Subsystem
  carrier signal : Sin  Frequency=348*2*pi  SampleTime=0
  Out1 : Outport
  wires:
  carrier signal/1 -> Balanced Modulator/2(Carrier Signal)
  Balanced Modulator/1(DSBSC) -> Analog Filter Design/1
  Analog Filter Design/1 -> Out1/1
  Input Signal/1 -> Balanced Modulator/1(Input Signal)

== system signal_tranmission/SSB Modulator63 ==
  Input Signal : Inport
  Analog Filter Design : dspfdesign/Analog Filter Design  method=Butterworth  filttype=Bandpass  N=4  Wlo=350*2*pi  Whi=354*2*pi  Rp=2  Rs=40
  Balanced Modulator : Subsystem
  carrier signal : Sin  Frequency=352*2*pi  SampleTime=0
  Out1 : Outport
  wires:
  carrier signal/1 -> Balanced Modulator/2(Carrier Signal)
  Balanced Modulator/1(DSBSC) -> Analog Filter Design/1
  Analog Filter Design/1 -> Out1/1
  Input Signal/1 -> Balanced Modulator/1(Input Signal)

== system signal_tranmission/SSB Modulator64 ==
  Input Signal : Inport
  Analog Filter Design : dspfdesign/Analog Filter Design  method=Butterworth  filttype=Bandpass  N=4  Wlo=354*2*pi  Whi=358*2*pi  Rp=2  Rs=40
  Balanced Modulator : Subsystem
  carrier signal : Sin  Frequency=356*2*pi  SampleTime=0
  Out1 : Outport
  wires:
  carrier signal/1 -> Balanced Modulator/2(Carrier Signal)
  Balanced Modulator/1(DSBSC) -> Analog Filter Design/1
  Analog Filter Design/1 -> Out1/1
  Input Signal/1 -> Balanced Modulator/1(Input Signal)

== system signal_tranmission/SSB Modulator65 ==
  Input Signal : Inport
  Analog Filter Design : dspfdesign/Analog Filter Design  method=Butterworth  filttype=Bandpass  N=4  Wlo=358*2*pi  Whi=362*2*pi  Rp=2  Rs=40
  Balanced Modulator : Subsystem
  carrier signal : Sin  Frequency=360*2*pi  SampleTime=0
  Out1 : Outport
  wires:
  carrier signal/1 -> Balanced Modulator/2(Carrier Signal)
  Balanced Modulator/1(DSBSC) -> Analog Filter Design/1
  Analog Filter Design/1 -> Out1/1
  Input Signal/1 -> Balanced Modulator/1(Input Signal)

== system signal_tranmission/SSB Modulator66 ==
  Input Signal : Inport
  Analog Filter Design : dspfdesign/Analog Filter Design  method=Butterworth  filttype=Bandpass  N=4  Wlo=362*2*pi  Whi=366*2*pi  Rp=2  Rs=40
  Balanced Modulator : Subsystem
  carrier signal : Sin  Frequency=364*2*pi  SampleTime=0
  Out1 : Outport
  wires:
  carrier signal/1 -> Balanced Modulator/2(Carrier Signal)
  Balanced Modulator/1(DSBSC) -> Analog Filter Design/1
  Analog Filter Design/1 -> Out1/1
  Input Signal/1 -> Balanced Modulator/1(Input Signal)

== system signal_tranmission/SSB Modulator67 ==
  Input Signal : Inport
  Analog Filter Design : dspfdesign/Analog Filter Design  method=Butterworth  filttype=Bandpass  N=4  Wlo=366*2*pi  Whi=370*2*pi  Rp=2  Rs=40
  Balanced Modulator : Subsystem
  carrier signal : Sin  Frequency=368*2*pi  SampleTime=0
  Out1 : Outport
  wires:
  carrier signal/1 -> Balanced Modulator/2(Carrier Signal)
  Balanced Modulator/1(DSBSC) -> Analog Filter Design/1
  Analog Filter Design/1 -> Out1/1
  Input Signal/1 -> Balanced Modulator/1(Input Signal)

== system signal_tranmission/SSB Modulator68 ==
  Input Signal : Inport
  Analog Filter Design : dspfdesign/Analog Filter Design  method=Butterworth  filttype=Bandpass  N=4  Wlo=370*2*pi  Whi=374*2*pi  Rp=2  Rs=40
  Balanced Modulator : Subsystem
  carrier signal : Sin  Frequency=372*2*pi  SampleTime=0
  Out1 : Outport
  wires:
  carrier signal/1 -> Balanced Modulator/2(Carrier Signal)
  Balanced Modulator/1(DSBSC) -> Analog Filter Design/1
  Analog Filter Design/1 -> Out1/1
  Input Signal/1 -> Balanced Modulator/1(Input Signal)

== system signal_tranmission/SSB Modulator69 ==
  Input Signal : Inport
  Analog Filter Design : dspfdesign/Analog Filter Design  method=Butterworth  filttype=Bandpass  N=4  Wlo=374*2*pi  Whi=378*2*pi  Rp=2  Rs=40
  Balanced Modulator : Subsystem
  carrier signal : Sin  Frequency=376*2*pi  SampleTime=0
  Out1 : Outport
  wires:
  carrier signal/1 -> Balanced Modulator/2(Carrier Signal)
  Balanced Modulator/1(DSBSC) -> Analog Filter Design/1
  Analog Filter Design/1 -> Out1/1
  Input Signal/1 -> Balanced Modulator/1(Input Signal)

== system signal_tranmission/SSB Modulator7 ==
  Input Signal : Inport
  Analog Filter Design : dspfdesign/Analog Filter Design  method=Butterworth  filttype=Bandpass  N=4  Wlo=126*2*pi  Whi=130*2*pi  Rp=2  Rs=40
  Balanced Modulator : Subsystem
  carrier signal : Sin  Frequency=128*2*pi  SampleTime=0
  Out1 : Outport
  wires:
  carrier signal/1 -> Balanced Modulator/2(Carrier Signal)
  Balanced Modulator/1(DSBSC) -> Analog Filter Design/1
  Analog Filter Design/1 -> Out1/1
  Input Signal/1 -> Balanced Modulator/1(Input Signal)

== system signal_tranmission/SSB Modulator70 ==
  Input Signal : Inport
  Analog Filter Design : dspfdesign/Analog Filter Design  method=Butterworth  filttype=Bandpass  N=4  Wlo=378*2*pi  Whi=382*2*pi  Rp=2  Rs=40
  Balanced Modulator : Subsystem
  carrier signal : Sin  Frequency=380*2*pi  SampleTime=0
  Out1 : Outport
  wires:
  carrier signal/1 -> Balanced Modulator/2(Carrier Signal)
  Balanced Modulator/1(DSBSC) -> Analog Filter Design/1
  Analog Filter Design/1 -> Out1/1
  Input Signal/1 -> Balanced Modulator/1(Input Signal)

== system signal_tranmission/SSB Modulator71 ==
  Input Signal : Inport
  Analog Filter Design : dspfdesign/Analog Filter Design  method=Butterworth  filttype=Bandpass  N=4  Wlo=382*2*pi  Whi=386*2*pi  Rp=2  Rs=40
  Balanced Modulator : Subsystem
  carrier signal : Sin  Frequency=384*2*pi  SampleTime=0
  Out1 : Outport
  wires:
  carrier signal/1 -> Balanced Modulator/2(Carrier Signal)
  Balanced Modulator/1(DSBSC) -> Analog Filter Design/1
  Analog Filter Design/1 -> Out1/1
  Input Signal/1 -> Balanced Modulator/1(Input Signal)

== system signal_tranmission/SSB Modulator72 ==
  Input Signal : Inport
  Analog Filter Design : dspfdesign/Analog Filter Design  method=Butterworth  filttype=Bandpass  N=4  Wlo=386*2*pi  Whi=390*2*pi  Rp=2  Rs=40
  Balanced Modulator : Subsystem
  carrier signal : Sin  Frequency=388*2*pi  SampleTime=0
  Out1 : Outport
  wires:
  carrier signal/1 -> Balanced Modulator/2(Carrier Signal)
  Balanced Modulator/1(DSBSC) -> Analog Filter Design/1
  Analog Filter Design/1 -> Out1/1
  Input Signal/1 -> Balanced Modulator/1(Input Signal)

== system signal_tranmission/SSB Modulator73 ==
  Input Signal : Inport
  Analog Filter Design : dspfdesign/Analog Filter Design  method=Butterworth  filttype=Bandpass  N=4  Wlo=390*2*pi  Whi=394*2*pi  Rp=2  Rs=40
  Balanced Modulator : Subsystem
  carrier signal : Sin  Frequency=392*2*pi  SampleTime=0
  Out1 : Outport
  wires:
  carrier signal/1 -> Balanced Modulator/2(Carrier Signal)
  Balanced Modulator/1(DSBSC) -> Analog Filter Design/1
  Analog Filter Design/1 -> Out1/1
  Input Signal/1 -> Balanced Modulator/1(Input Signal)

== system signal_tranmission/SSB Modulator74 ==
  Input Signal : Inport
  Analog Filter Design : dspfdesign/Analog Filter Design  method=Butterworth  filttype=Bandpass  N=4  Wlo=394*2*pi  Whi=398*2*pi  Rp=2  Rs=40
  Balanced Modulator : Subsystem
  carrier signal : Sin  Frequency=396*2*pi  SampleTime=0
  Out1 : Outport
  wires:
  carrier signal/1 -> Balanced Modulator/2(Carrier Signal)
  Balanced Modulator/1(DSBSC) -> Analog Filter Design/1
  Analog Filter Design/1 -> Out1/1
  Input Signal/1 -> Balanced Modulator/1(Input Signal)

== system signal_tranmission/SSB Modulator75 ==
  Input Signal : Inport
  Analog Filter Design : dspfdesign/Analog Filter Design  method=Butterworth  filttype=Bandpass  N=4  Wlo=398*2*pi  Whi=402*2*pi  Rp=2  Rs=40
  Balanced Modulator : Subsystem
  carrier signal : Sin  Frequency=400*2*pi  SampleTime=0
  Out1 : Outport
  wires:
  carrier signal/1 -> Balanced Modulator/2(Carrier Signal)
  Balanced Modulator/1(DSBSC) -> Analog Filter Design/1
  Analog Filter Design/1 -> Out1/1
  Input Signal/1 -> Balanced Modulator/1(Input Signal)

== system signal_tranmission/SSB Modulator76 ==
  Input Signal : Inport
  Analog Filter Design : dspfdesign/Analog Filter Design  method=Butterworth  filttype=Bandpass  N=4  Wlo=402*2*pi  Whi=406*2*pi  Rp=2  Rs=40
  Balanced Modulator : Subsystem
  carrier signal : Sin  Frequency=404*2*pi  SampleTime=0
  Out1 : Outport
  wires:
  carrier signal/1 -> Balanced Modulator/2(Carrier Signal)
  Balanced Modulator/1(DSBSC) -> Analog Filter Design/1
  Analog Filter Design/1 -> Out1/1
  Input Signal/1 -> Balanced Modulator/1(Input Signal)

== system signal_tranmission/SSB Modulator77 ==
  Input Signal : Inport
  Analog Filter Design : dspfdesign/Analog Filter Design  method=Butterworth  filttype=Bandpass  N=4  Wlo=406*2*pi  Whi=410*2*pi  Rp=2  Rs=40
  Balanced Modulator : Subsystem
  carrier signal : Sin  Frequency=408*2*pi  SampleTime=0
  Out1 : Outport
  wires:
  carrier signal/1 -> Balanced Modulator/2(Carrier Signal)
  Balanced Modulator/1(DSBSC) -> Analog Filter Design/1
  Analog Filter Design/1 -> Out1/1
  Input Signal/1 -> Balanced Modulator/1(Input Signal)

== system signal_tranmission/SSB Modulator78 ==
  Input Signal : Inport
  Analog Filter Design : dspfdesign/Analog Filter Design  method=Butterworth  filttype=Bandpass  N=4  Wlo=410*2*pi  Whi=414*2*pi  Rp=2  Rs=40
  Balanced Modulator : Subsystem
  carrier signal : Sin  Frequency=412*2*pi  SampleTime=0
  Out1 : Outport
  wires:
  carrier signal/1 -> Balanced Modulator/2(Carrier Signal)
  Balanced Modulator/1(DSBSC) -> Analog Filter Design/1
  Analog Filter Design/1 -> Out1/1
  Input Signal/1 -> Balanced Modulator/1(Input Signal)

== system signal_tranmission/SSB Modulator79 ==
  Input Signal : Inport
  Analog Filter Design : dspfdesign/Analog Filter Design  method=Butterworth  filttype=Bandpass  N=4  Wlo=414*2*pi  Whi=418*2*pi  Rp=2  Rs=40
  Balanced Modulator : Subsystem
  carrier signal : Sin  Frequency=416*2*pi  SampleTime=0
  Out1 : Outport
  wires:
  carrier signal/1 -> Balanced Modulator/2(Carrier Signal)
  Balanced Modulator/1(DSBSC) -> Analog Filter Design/1
  Analog Filter Design/1 -> Out1/1
  Input Signal/1 -> Balanced Modulator/1(Input Signal)

== system signal_tranmission/SSB Modulator8 ==
  Input Signal : Inport
  Analog Filter Design : dspfdesign/Analog Filter Design  method=Butterworth  filttype=Bandpass  N=4  Wlo=130*2*pi  Whi=134*2*pi  Rp=2  Rs=40
  Balanced Modulator : Subsystem
  carrier signal : Sin  Frequency=132*2*pi  SampleTime=0
  Out1 : Outport
  wires:
  carrier signal/1 -> Balanced Modulator/2(Carrier Signal)
  Balanced Modulator/1(DSBSC) -> Analog Filter Design/1
  Analog Filter Design/1 -> Out1/1
  Input Signal/1 -> Balanced Modulator/1(Input Signal)

== system signal_tranmission/SSB Modulator80 ==
  Input Signal : Inport
  Analog Filter Design : dspfdesign/Analog Filter Design  method=Butterworth  filttype=Bandpass  N=4  Wlo=418*2*pi  Whi=422*2*pi  Rp=2  Rs=40
  Balanced Modulator : Subsystem
  carrier signal : Sin  Frequency=420*2*pi  SampleTime=0
  Out1 : Outport
  wires:
  carrier signal/1 -> Balanced Modulator/2(Carrier Signal)
  Balanced Modulator/1(DSBSC) -> Analog Filter Design/1
  Analog Filter Design/1 -> Out1/1
  Input Signal/1 -> Balanced Modulator/1(Input Signal)

== system signal_tranmission/SSB Modulator81 ==
  Input Signal : Inport
  Analog Filter Design : dspfdesign/Analog Filter Design  method=Butterworth  filttype=Bandpass  N=4  Wlo=422*2*pi  Whi=426*2*pi  Rp=2  Rs=40
  Balanced Modulator : Subsystem
  carrier signal : Sin  Frequency=424*2*pi  SampleTime=0
  Out1 : Outport
  wires:
  carrier signal/1 -> Balanced Modulator/2(Carrier Signal)
  Balanced Modulator/1(DSBSC) -> Analog Filter Design/1
  Analog Filter Design/1 -> Out1/1
  Input Signal/1 -> Balanced Modulator/1(Input Signal)

== system signal_tranmission/SSB Modulator82 ==
  Input Signal : Inport
  Analog Filter Design : dspfdesign/Analog Filter Design  method=Butterworth  filttype=Bandpass  N=4  Wlo=426*2*pi  Whi=430*2*pi  Rp=2  Rs=40
  Balanced Modulator : Subsystem
  carrier signal : Sin  Frequency=428*2*pi  SampleTime=0
  Out1 : Outport
  wires:
  carrier signal/1 -> Balanced Modulator/2(Carrier Signal)
  Balanced Modulator/1(DSBSC) -> Analog Filter Design/1
  Analog Filter Design/1 -> Out1/1
  Input Signal/1 -> Balanced Modulator/1(Input Signal)

== system signal_tranmission/SSB Modulator83 ==
  Input Signal : Inport
  Analog Filter Design : dspfdesign/Analog Filter Design  method=Butterworth  filttype=Bandpass  N=4  Wlo=430*2*pi  Whi=434*2*pi  Rp=2  Rs=40
  Balanced Modulator : Subsystem
  carrier signal : Sin  Frequency=432*2*pi  SampleTime=0
  Out1 : Outport
  wires:
  carrier signal/1 -> Balanced Modulator/2(Carrier Signal)
  Balanced Modulator/1(DSBSC) -> Analog Filter Design/1
  Analog Filter Design/1 -> Out1/1
  Input Signal/1 -> Balanced Modulator/1(Input Signal)

== system signal_tranmission/SSB Modulator84 ==
  Input Signal : Inport
  Analog Filter Design : dspfdesign/Analog Filter Design  method=Butterworth  filttype=Bandpass  N=4  Wlo=434*2*pi  Whi=438*2*pi  Rp=2  Rs=40
  Balanced Modulator : Subsystem
  carrier signal : Sin  Frequency=436*2*pi  SampleTime=0
  Out1 : Outport
  wires:
  carrier signal/1 -> Balanced Modulator/2(Carrier Signal)
  Balanced Modulator/1(DSBSC) -> Analog Filter Design/1
  Analog Filter Design/1 -> Out1/1
  Input Signal/1 -> Balanced Modulator/1(Input Signal)
